simulink model "simulink_caso1_digital"  (R2023a)
settings: Solver=VariableStepAuto  StartTime=0.0  StopTime=6  MaxStep=0.001  MinStep=0.0001  RelTol=1e-3  EnableMultiTasking=on
undefined symbols (not defined in the file): Ad, Aestd, Bd, Bestd, Cd, Cestd, Dd, Destd, K0d, Kd, Ts
settings Model: Creator=54115  LastModifiedBy=Agustin
settings SolverCC: AlgebraicLoopSolver=TrustRegion
settings DataIOCC: ReturnWorkspaceOutputs=off
settings OptimizationCC: LifeSpan=inf
settings DebuggingCC: UnconnectedInputMsg=warning  UnconnectedOutputMsg=warning  UnconnectedLineMsg=warning  SFUnexpectedBacktrackingDiag=warning  SFNoUnconditionalDefaultTransitionDiag=warning  ArithmeticOperatorsInVariantConditions=warning
settings ModelReferenceCC: EnableRefExpFcnMdlSchedulingChecks=on
settings SFSimCC: SimUseLocalCustomCode=off  CustomCodeUndefinedFunction=UseInterfaceOnly
settings RTWCC: RTWUseLocalCustomCode=off
settings CodeAppCC: StateflowObjectComments=on
settings GRTTargetCC: TargetLangStandard=C89/C90 (ANSI)
settings ConfigComp: CovMetricSettings=dw  CovSaveCumulativeToWorkspaceVar=on  CovSaveSingleToWorkspaceVar=on  CovExternalEMLEnable=off

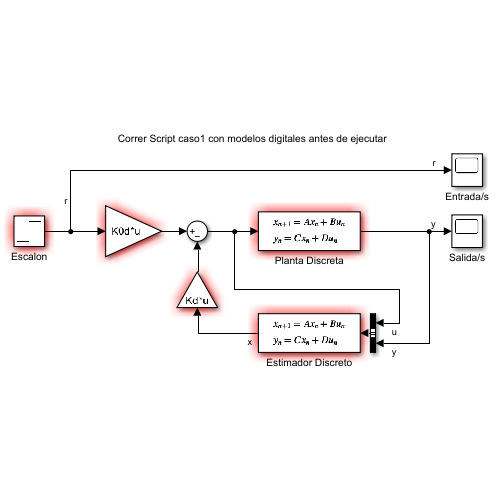
[thumbnail: Simulink's stored preview of the top-level diagram]
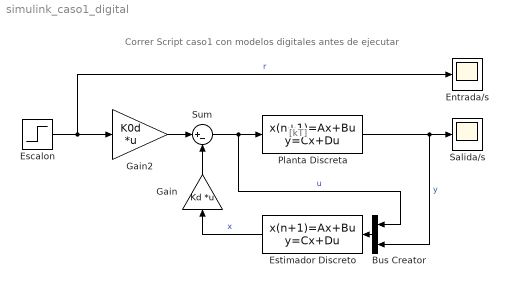
== system simulink_caso1_digital ==
  note: [kT]
  note: Correr Script caso1 con modelos digitales antes de ejecutar
  Bus Creator : BusCreator  Inputs=2
  Entrada/s : Scope
  Escalon : Step  SampleTime=Ts
  Estimador Discreto : DiscreteStateSpace  A=Aestd  B=Bestd  C=Cestd  D=Destd  SampleTime=Ts
  Gain : Gain  Gain=Kd  Multiplication=Matrix(K*u)
  Gain2 : Gain  Gain=K0d  Multiplication=Matrix(K*u)
  Planta Discreta : DiscreteStateSpace  A=Ad  B=Bd  C=Cd  D=Dd  SampleTime=Ts
  Salida/s : Scope
  Sum : Sum  Inputs=|+-
  wires:
  Estimador Discreto/1 -> Gain/1  "x"
  Bus Creator/1 -> Estimador Discreto/1
  Gain2/1 -> Sum/1
  Gain/1 -> Sum/2
  Sum/1 -> Planta Discreta/1, Bus Creator/1  "u"
  Planta Discreta/1 -> Salida/s/1, Bus Creator/2  "y"
  Escalon/1 -> Entrada/s/1, Gain2/1  "r"
